simulink model "active_Balancing1"  (R2021a)
settings: Solver=VariableStepAuto  StartTime=0.0  StopTime=10000  RelTol=1e-3
undefined symbols (not defined in the file): Ion, Lithium
libraries: spsSeriesRLCBranchLib x6, spsMosfetLib x6, spsBatteryLib x4, spsVoltageMeasurementLib x1, spspowerguiLib x1
settings Model: PacingRate=50  Creator=Navadeep  LastModifiedBy=Navadeep

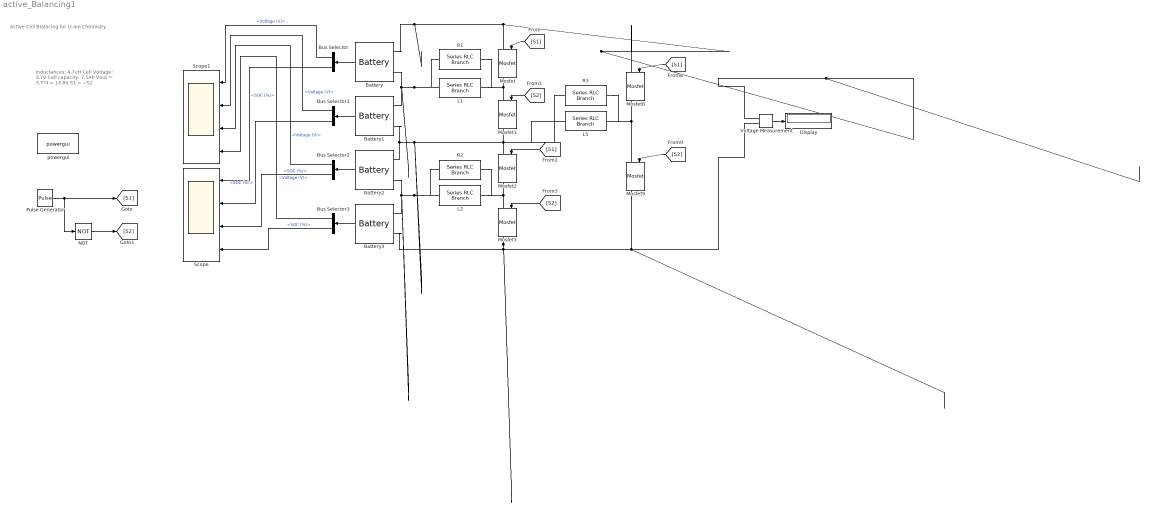
== system active_Balancing1 ==
  note: Active Cell Blalacing for Li-Ion Chemistry
  note: Inductances: 4.7uH
      | Cell Voltage: 3.7V
      | Cell capacity: 7.5Ah
      | Vout = 3.7*4 = 14.8V
      |
      | S1 = ~S2
  Battery : spsBatteryLib/Battery  BatType=Lithium-Ion  ShowTempParam=off  ThermalPreset=no  ShowAgeParam=off  NomV=3.7  NomQ=7.5  SOC=80  Batt_Tr=30  PresetModel=on  MaxQ=7.5  MinV=2.775  FullV=4.3068  Dis_rate=3.2609  R=0.0049333  Normal_OP=6.7826  expZone="[3.9974     0.36848]"  current=[6.5 13 32.5]  Units=Time  Tci=20  NomT=20  T2=-30  MaxQ2=4.8  FullV2=7.1  Normal_OP2=5.655  expZone2="[6.58           1]"  Rca=0.6  ti=2000  Dp=0  Neq0=0  Tsim=1e6  Ta1=25  Qeol=5.4*0.9  Reol=0.013333*1.2  Char_age=[2.3478, 3]  Dis_age=[2.3478, 10]  N1=1500  N2=10500  N3=1000  N4=1400  Ta2=45  N5=950
  Battery1 : spsBatteryLib/Battery  BatType=Lithium-Ion  ShowTempParam=off  ThermalPreset=no  ShowAgeParam=off  NomV=3.7  NomQ=7.5  SOC=95  Batt_Tr=30  PresetModel=on  MaxQ=7.5  MinV=2.775  FullV=4.3068  Dis_rate=3.2609  R=0.0049333  Normal_OP=6.7826  expZone="[3.9974     0.36848]"  current=[6.5 13 32.5]  Units=Time  Tci=20  NomT=20  T2=-30  MaxQ2=4.8  FullV2=7.1  Normal_OP2=5.655  expZone2="[6.58           1]"  Rca=0.6  ti=2000  Dp=0  Neq0=0  Tsim=1e6  Ta1=25  Qeol=5.4*0.9  Reol=0.013333*1.2  Char_age=[2.3478, 3]  Dis_age=[2.3478, 10]  N1=1500  N2=10500  N3=1000  N4=1400  Ta2=45  N5=950
  Battery2 : spsBatteryLib/Battery  BatType=Lithium-Ion  ShowTempParam=off  ThermalPreset=no  ShowAgeParam=off  NomV=3.7  NomQ=7.5  SOC=70  Batt_Tr=30  PresetModel=on  MaxQ=7.5  MinV=2.775  FullV=4.3068  Dis_rate=3.2609  R=0.0049333  Normal_OP=6.7826  expZone="[3.9974     0.36848]"  current=[6.5 13 32.5]  Units=Time  Tci=20  NomT=20  T2=-30  MaxQ2=4.8  FullV2=7.1  Normal_OP2=5.655  expZone2="[6.58           1]"  Rca=0.6  ti=2000  Dp=0  Neq0=0  Tsim=1e6  Ta1=25  Qeol=5.4*0.9  Reol=0.013333*1.2  Char_age=[2.3478, 3]  Dis_age=[2.3478, 10]  N1=1500  N2=10500  N3=1000  N4=1400  Ta2=45  N5=950
  Battery3 : spsBatteryLib/Battery  BatType=Lithium-Ion  ShowTempParam=off  ThermalPreset=no  ShowAgeParam=off  NomV=3.7  NomQ=7.5  SOC=85  Batt_Tr=30  PresetModel=on  MaxQ=7.5  MinV=2.775  FullV=4.3068  Dis_rate=3.2609  R=0.0049333  Normal_OP=6.7826  expZone="[3.9974     0.36848]"  current=[6.5 13 32.5]  Units=Time  Tci=20  NomT=20  T2=-30  MaxQ2=4.8  FullV2=7.1  Normal_OP2=5.655  expZone2="[6.58           1]"  Rca=0.6  ti=2000  Dp=0  Neq0=0  Tsim=1e6  Ta1=25  Qeol=5.4*0.9  Reol=0.013333*1.2  Char_age=[2.3478, 3]  Dis_age=[2.3478, 10]  N1=1500  N2=10500  N3=1000  N4=1400  Ta2=45  N5=950
  Bus Selector{,1..3} (4 alike) : BusSelector  OutputSignals=Voltage (V),Current (A),SOC (%)
  Display : Display
  L1 : spsSeriesRLCBranchLib/Series RLC Branch  LConnTagsString=__new0  RConnTagsString=__new0  BranchType=L  Resistance=1  Inductance=4.7e-6  SetiL0=off  InitialCurrent=0  Capacitance=1e-6  Setx0=off  InitialVoltage=0  Measurements=None
  L2 : spsSeriesRLCBranchLib/Series RLC Branch  LConnTagsString=__new0  RConnTagsString=__new0  BranchType=L  Resistance=1  Inductance=4.7e-6  SetiL0=off  InitialCurrent=0  Capacitance=1e-6  Setx0=off  InitialVoltage=0  Measurements=None
  L5 : spsSeriesRLCBranchLib/Series RLC Branch  LConnTagsString=__new0  RConnTagsString=__new0  BranchType=L  Resistance=1  Inductance=4.7e-6  SetiL0=off  InitialCurrent=0  Capacitance=1e-6  Setx0=off  InitialVoltage=0  Measurements=None
  Mosfet{,1..3,8..9} (6 alike) : spsMosfetLib/Mosfet  Ron=0.1  Lon=0  Rd=0.01  Vfd=0  IC=0  Rs=1e5  Cs=inf  Measurements=on
  NOT : Logic  Operator=NOT  IconShape=distinctive  AllPortsSameDT=off  OutDataTypeStr=boolean
  Pulse Generator : DiscretePulseGenerator  PulseType=Time based  Period=1e-3  PulseWidth=50
  R1 : spsSeriesRLCBranchLib/Series RLC Branch  LConnTagsString=__new0  RConnTagsString=__new0  BranchType=R  Resistance=2000  Inductance=1e-3  SetiL0=off  InitialCurrent=0  Capacitance=1e-6  Setx0=off  InitialVoltage=0  Measurements=None
  R2 : spsSeriesRLCBranchLib/Series RLC Branch  LConnTagsString=__new0  RConnTagsString=__new0  BranchType=R  Resistance=2000  Inductance=1e-3  SetiL0=off  InitialCurrent=0  Capacitance=1e-6  Setx0=off  InitialVoltage=0  Measurements=None
  R3 : spsSeriesRLCBranchLib/Series RLC Branch  LConnTagsString=__new0  RConnTagsString=__new0  BranchType=R  Resistance=2000  Inductance=1e-3  SetiL0=off  InitialCurrent=0  Capacitance=1e-6  Setx0=off  InitialVoltage=0  Measurements=None
  Scope : Scope  NumInputPorts=4
  Scope1 : Scope  NumInputPorts=4
  Voltage Measurement : spsVoltageMeasurementLib/Voltage Measurement  PhasorSimulation=off  OutputType=Complex  PSBequivalent=0
  powergui : spspowerguiLib/powergui  Priority=1  SimulationMode=Discrete  SampleTime=5e-2  frequency=60  Iterations=50  frequencyindice=0  Pbase=100e6  ErrMax=1e-4  UnitsV=kV  UnitsW=MW  buscounter=0  FunctionMessages=off  echomessages=off  EnableUseOfTLC=off  CurrentSourceSwitches=off  DisableSnubberDevices=off  DisableRonSwitches=off  DisableVfSwitches=off  DisplayEquations=off  AutomaticDiscreteSolvers=off  SolverType=Tustin/Backward Euler (TBE)  Interpol=off  ExternalGateDelay=off  methode=off  Ts=100  x0status=blocks  SPID=on  SwTol=0  HookPort=off  NonlinearTolerance=1e-4  nMaxIteration=100  ContinueOnMaxIteration=off  RestoreLinks=warning  ResistiveCurrentMeasurement=off  Frange=[0:2:500]  Ylog=off  Xlog=on  ShowGrid=off  save=off  variable=ZData  structure=0  ZoomFFT=off  StartTime=0.0  cycles=1  DisplayStyle=1  fundamental=60  FreqAxis=off  MaxFrequency=1000  frequencyindicesteady=1  RmsSteady=1  display=off
  wires:
  [S1] -> Mosfet/1
  [S2] -> Mosfet1/1
  [S1] -> Mosfet2/1
  [S2] -> Mosfet3/1
  [S2] -> Mosfet9/1
  [S1] -> Mosfet8/1
  Pulse Generator/1 -> [S1], NOT/1
  Battery/1 -> Bus Selector/1
  Battery1/1 -> Bus Selector1/1
  Battery3/1 -> Bus Selector3/1
  Battery2/1 -> Bus Selector2/1
  Bus Selector/3 -> Scope/1  "<SOC (%)>"
  Bus Selector1/3 -> Scope/2  "<SOC (%)>"
  Bus Selector2/3 -> Scope/3  "<SOC (%)>"
  Bus Selector3/3 -> Scope/4  "<SOC (%)>"
  Bus Selector/1 -> Scope1/1  "<Voltage (V)>"
  Bus Selector1/1 -> Scope1/2  "<Voltage (V)>"
  Bus Selector2/1 -> Scope1/3  "<Voltage (V)>"
  NOT/1 -> [S2]
  Voltage Measurement/1 -> Display/1
  Bus Selector3/1 -> Scope1/4  "<Voltage (V)>"
  connections:
  Battery/LConn2 -- R1/RConn1 -- L1/LConn1 -- Battery1/LConn1
  Mosfet2/LConn1 -- R3/RConn1 -- L5/LConn1 -- Mosfet1/RConn1 -- Battery1/LConn2 -- Battery2/LConn1
  Battery2/LConn2 -- R2/RConn1 -- L2/LConn1 -- Battery3/LConn1
  Mosfet3/RConn1 -- Battery3/LConn2 -- Voltage Measurement/LConn2 -- Mosfet9/RConn1
  Mosfet3/LConn1 -- R2/LConn1 -- L2/RConn1 -- Mosfet2/RConn1
  Mosfet1/LConn1 -- R1/LConn1 -- L1/RConn1 -- Mosfet/RConn1
  Battery/LConn1 -- Voltage Measurement/LConn1 -- Mosfet8/LConn1 -- Mosfet/LConn1
  Mosfet9/LConn1 -- R3/LConn1 -- L5/RConn1 -- Mosfet8/RConn1
